simulink model "zad2"  (R2016a)
settings: Solver=VariableStepAuto  StartTime=0.0  StopTime=100  MaxStep=2^-7  RelTol=1e-3
settings Model: Creator=sk42595  LastModifiedBy=sk42595

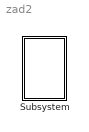
== system zad2 ==
  Subsystem : Subsystem  mask{k=1, m=10, l=3, g=10, fi0=90}

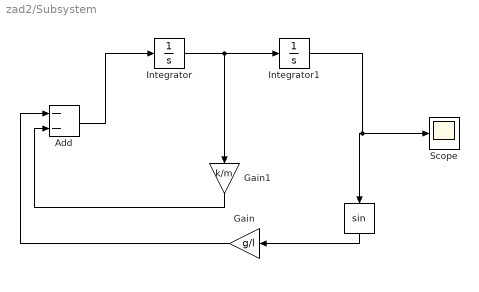
== system zad2/Subsystem ==
  " " : Trigonometry
  Add : Sum  Inputs=--
  Gain : Gain  Gain=g/l
  Gain1 : Gain  Gain=k/m
  Integrator : Integrator
  Integrator1 : Integrator  InitialCondition=(pi * fi0) / 180
  Scope : Scope
  wires:
  Integrator1/1 -> Scope/1, " "/1
  Gain/1 -> Add/1
  " "/1 -> Gain/1
  Gain1/1 -> Add/2
  Add/1 -> Integrator/1
  Integrator/1 -> Integrator1/1, Gain1/1
